simulink model "simulation"  (R2020a)
settings: Solver=ode3  StartTime=0.0  StopTime=20.0  FixedStep=Ts  RelTol=1e-3
values from neighbouring files (symbols this model uses):
  L = 1    [BinomeName.m]    (also in bifurcation_diagram.m; derivee.m = input(5))
  R = list_R(i)    [BinomeName.m]    (also in bifurcation_diagram.m; derivee.m = input(6))
  X0 = [0 ; 0 ; 0 ; 0]    [BinomeName.m]    (also in bifurcation_diagram.m)
undefined symbols (not defined in the file or in its folder): derivee
libraries: simulink x4
settings Model: Creator=paupa  LastModifiedBy=paupa

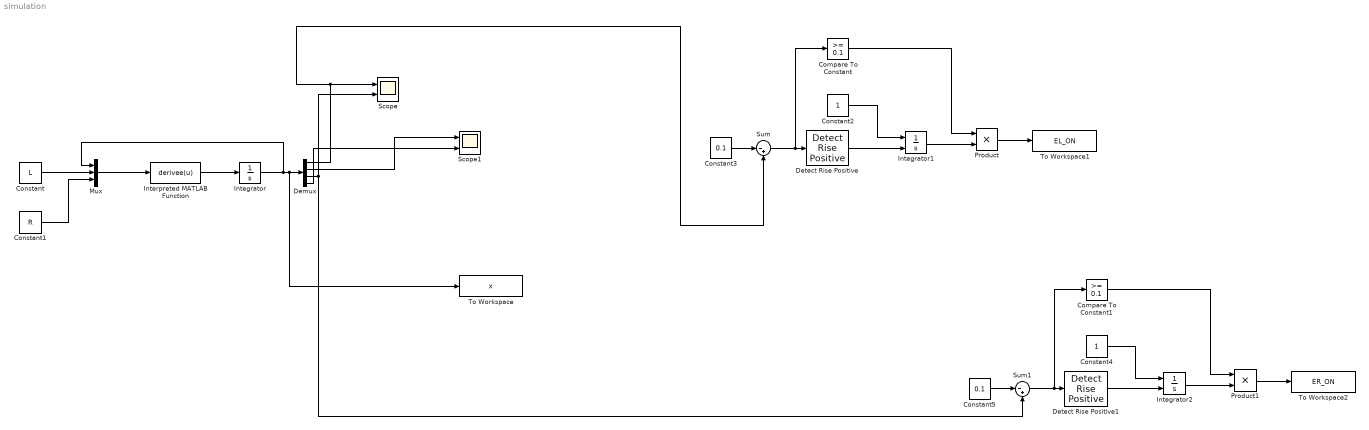
== system simulation ==
  Compare To Constant : simulink/Logic and Bit Operations/Compare To Constant  relop=>=  const=0.1  OutDataTypeStr=boolean
  Compare To Constant1 : simulink/Logic and Bit Operations/Compare To Constant  relop=>=  const=0.1  OutDataTypeStr=boolean
  Constant : Constant  Value=L
  Constant1 : Constant  Value=R
  Constant2 : Constant
  Constant3 : Constant  Value=0.1
  Constant4 : Constant
  Constant5 : Constant  Value=0.1
  Demux : Demux
  Detect Rise Positive : simulink/Logic and Bit Operations/Detect Rise Positive  vinit=0  OutDataTypeStr=boolean
  Detect Rise Positive1 : simulink/Logic and Bit Operations/Detect Rise Positive  vinit=0  OutDataTypeStr=boolean
  Integrator : Integrator  InitialCondition=X0
  Integrator1 : Integrator  ExternalReset=rising
  Integrator2 : Integrator  ExternalReset=rising
  Interpreted MATLAB Function : MATLABFcn  MATLABFcn=derivee(u)  OutputDimensions=4  Output1D=off
  Mux : Mux  Inputs=3
  Product : Product
  Product1 : Product
  Scope : Scope  NumInputPorts=2
  Scope1 : Scope  NumInputPorts=2
  Sum : Sum  Inputs=|-+
  Sum1 : Sum  Inputs=|-+
  To Workspace : ToWorkspace  VariableName=x  SaveFormat=Timeseries  SampleTime=-1
  To Workspace1 : ToWorkspace  VariableName=EL_ON  SaveFormat=Structure With Time  SampleTime=-1
  To Workspace2 : ToWorkspace  VariableName=ER_ON  SaveFormat=Structure With Time  SampleTime=-1
  wires:
  Interpreted MATLAB Function/1 -> Integrator/1
  Integrator/1 -> Mux/1, To Workspace/1, Demux/1
  Demux/3 -> Sum1/2, Scope/2
  Demux/2 -> Scope1/1
  Demux/4 -> Scope1/2
  Constant/1 -> Mux/2
  Constant1/1 -> Mux/3
  Mux/1 -> Interpreted MATLAB Function/1
  Compare To Constant/1 -> Product/1
  Sum/1 -> Compare To Constant/1, Detect Rise Positive/1
  Integrator1/1 -> Product/2
  Demux/1 -> Scope/1, Sum/2
  Constant3/1 -> Sum/1
  Constant2/1 -> Integrator1/1
  Detect Rise Positive/1 -> Integrator1/2
  Product/1 -> To Workspace1/1
  Integrator2/1 -> Product1/2
  Constant4/1 -> Integrator2/1
  Detect Rise Positive1/1 -> Integrator2/2
  Compare To Constant1/1 -> Product1/1
  Sum1/1 -> Compare To Constant1/1, Detect Rise Positive1/1
  Constant5/1 -> Sum1/1
  Product1/1 -> To Workspace2/1
